simulink model "Copy_of_simulink_ros"  (R2022b)
settings: Solver=FixedStepAuto  StartTime=0.0  StopTime=10.0  FixedStep=0.01  RelTol=1e-3
libraries: robotlib x5
settings Model: Creator=pico  LastModifiedBy=pico

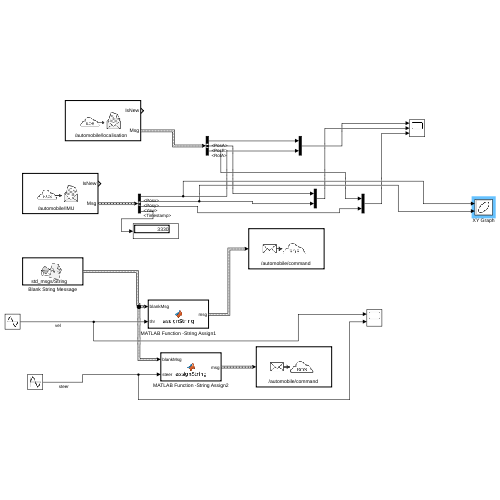
[thumbnail: Simulink's stored preview of the top-level diagram]
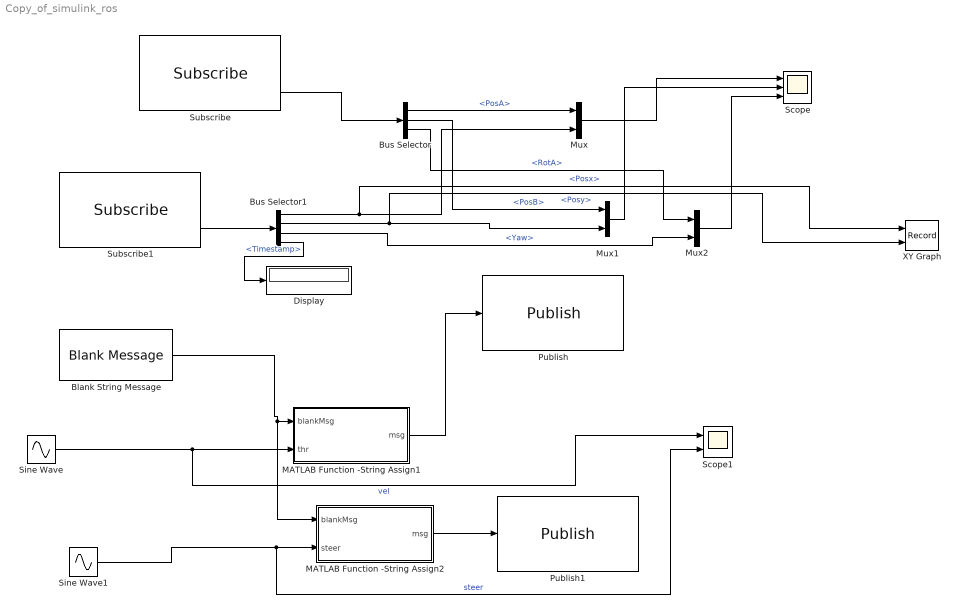
== system Copy_of_simulink_ros ==
  Blank String Message : robotlib/Blank Message  messageClass=Message  entityType=std_msgs/String  messageType=std_msgs/String  SampleTime=inf  legacyBusStruct=off
  Bus Selector : BusSelector  OutputSignals=PosA,PosB,RotA
  Bus Selector1 : BusSelector  OutputSignals=Posx,Posy,Yaw,Timestamp
  Display : Display
  MATLAB Function -String Assign1 : MATLAB Function  TreatAsAtomicUnit=on
  MATLAB Function -String Assign2 : MATLAB Function  TreatAsAtomicUnit=on
  Mux : Mux  Inputs=2
  Mux1 : Mux  Inputs=2
  Mux2 : Mux  Inputs=2
  Publish : robotlib/Publish  topicSource=Select from ROS network  topic=/automobile/command  messageType=std_msgs/String  legacyBusStruct=off  messageQueueLength=1
      settings: LibrarySourceBlock=roslib/ROS/Publish
  Publish1 : robotlib/Publish  topicSource=Select from ROS network  topic=/automobile/command  messageType=std_msgs/String  legacyBusStruct=off  messageQueueLength=1
      settings: LibrarySourceBlock=roslib/ROS/Publish
  Scope : Scope  NumInputPorts=3
  Scope1 : Scope  NumInputPorts=2
  Sine Wave : Sin  Amplitude=2.5  Bias=3  SampleTime=0
  Sine Wave1 : Sin  Amplitude=5  Frequency=2  SampleTime=0
  Subscribe : robotlib/Subscribe  topicSource=Select from ROS network  topic=/automobile/localisation  messageType=utils/localisation  SampleTime=-1  legacyBusStruct=off  messageQueueLength=1
      settings: LibrarySourceBlock=roslib/ROS/Subscribe
  Subscribe1 : robotlib/Subscribe  topicSource=Select from ROS network  topic=/automobile/IMU  messageType=utils/IMU  SampleTime=-1  legacyBusStruct=off  messageQueueLength=1
      settings: LibrarySourceBlock=roslib/ROS/Subscribe
  XY Graph : Record  FileSettingsInternal="{\"entries\":[{\"content\":{\"excelSettings\":{\"content\":{},\"type\":\"Streamout.ExcelSettings\"}},\"type\":\"Streamout.FileSettingStorage\",\"uuid\":\"e51b2920-8d42-452a-b452-2900fad765ce\"}],\"packageUris\":[\"http://schema.mathworks.com/mf0/streamout_blocks/R2020a\"],\"version\":\"1.0\"}"  Layout=[1 1]  SignalsInternal="{\"entries\":[{\"content\":{\"signals\":[{\"content\":{\"blockPath\":[\"simulink_ros/XY Graph\"],\"channel\":[],\"dimensions\":[1],\"domain\":\"simulink_ros/XY Graph\",\"lineColor\":\"#a2142f\",\"plots\":[1],\"port\":1,\"sid\":[\"\"],\"signalID\":1728,\"signalName\":\"<Posx>\"},\"type\":\"RecordBlkView.Signal\",\"uuid\":\"d8332a72-887d-4bf0-9569-057e20747bf9\"},{\"content\":{\"blockPath\":[\"simulink_ros/XY Graph\"],\"channel\":[],\"dimensions\":[1],\"domain\":\"simulink_ros/XY Graph\",\"lineColor\":\"#139fff\",\"plots\":[1],\"port\":2,\"sid\":[\"\"],\"signalID\":1732,\"signalName\":\"<Posy>\"},\"type\":\"RecordBlkView.Signal\",\"uuid\":\"ee58e5d7-22af-4a01-a3d3-c94aa3d0d7b0\"}]},\"type\":\"RecordBlkView.InputSignals\",\"uuid\":\"e0c6eb76-3918-4986-a988-b23fbc1792f6\"}],\"packageUris\":[\"http://schema.mathworks.com/mf0/streamout_blocks/R2020a\"],\"version\":\"1.0\"}"  VisualizationBindings="{\"xyplotplugin\":{\"info\":[{\"series\":[{\"bindingParametersList\":[{\"parameter\":\"X-Axis\",\"signalID\":1728,\"signalName\":\"<Posx>\"},{\"parameter\":\"Y-Axis\",\"signalID\":1732,\"signalName\":\"<Posy>\"}],\"seriesID\":33123}],\"subplotID\":1}]}}"  CompatibilityTag=XY
  wires:
  Subscribe/2 -> Bus Selector/1
  Bus Selector/1 -> Mux/1  "<PosA>"
  Blank String Message/1 -> MATLAB Function -String Assign2/1(blankMsg), MATLAB Function -String Assign1/1(blankMsg)
  MATLAB Function -String Assign1/1(msg) -> Publish/1
  Sine Wave/1 -> Scope1/1, MATLAB Function -String Assign1/2(thr)  "vel"
  MATLAB Function -String Assign2/1(msg) -> Publish1/1
  Sine Wave1/1 -> Scope1/2, MATLAB Function -String Assign2/2(steer)  "steer"
  Subscribe1/2 -> Bus Selector1/1
  Bus Selector1/1 -> XY Graph/1, Mux/2  "<Posx>"
  Bus Selector1/2 -> XY Graph/2, Mux1/2  "<Posy>"
  Mux/1 -> Scope/1
  Bus Selector/2 -> Mux1/1  "<PosB>"
  Mux1/1 -> Scope/2
  Bus Selector1/3 -> Mux2/2  "<Yaw>"
  Bus Selector/3 -> Mux2/1  "<RotA>"
  Mux2/1 -> Scope/3
  Bus Selector1/4 -> Display/1  "<Timestamp>"

== matlab function Copy_of_simulink_ros/MATLAB Function -String Assign2 ==
  data: blankMsg input; msg output Bus: SL_Bus_simulink_ros_std_msgs_String; steer input
function msg = assignString(blankMsg,steer)
% assignString - Assign a string in a ROS message
%
% MSG = assignString(blankMsg) assigns a known string value to a 
%  string field in a ROS message, and outputs the updated ROS message.
%
%  blankMsg (input): A bus for a 'std_msgs/String' message. This is 
%      used to initialize the output. 
%  msg (output): A bus for a 'std_msgs/String' message, with the Data 
%      field set to a string.

%   Copyright 2015 The MathWorks, Inc.
%#codegen

% Note: The datatype of 'msg' has been explicitly set to the appropriate 
% Simulink bus type ("Bus: SL_Bus_robotROSMessageUsageExample_std_msgs_String"). 
%
% If the model name is changed, the datatype needs to be changed as well:
%   1) Click "Edit Data" in the Editor toolstrip to open "Ports and Data Manager"
%   2) Select "msg". From the "Type" dropdown, select "--- Refresh data types ---"
%   3) Set datatype to "Bus: SL_Bus_<modelname>_std_msgs_String"
    
% stringToAssign = 'information';
steer_string = sprintf('%.1f',steer);
% "{\"action\": \"1\", \"speed\": -0.1}"
stringToAssign = ['{"action": "2", "steerAngle": ',steer_string,'}'];%['action\', '1', 'speed',u];

msg = blankMsg;

% msg (std_msgs/String) consists of
%           Data : array of type uint8
%   Data_SL_Info : struct with fields CurrentLength, ReceivedLength
strLength = length(stringToAssign);
msg.Data(1:strLength) = uint8(stringToAssign);
msg.Data_SL_Info.CurrentLength = uint32(strLength);

== matlab function Copy_of_simulink_ros/MATLAB Function -String Assign1 ==
  data: blankMsg input; msg output Bus: SL_Bus_simulink_ros_std_msgs_String; thr input
function msg = assignString(blankMsg,thr)
% assignString - Assign a string in a ROS message
%
% MSG = assignString(blankMsg) assigns a known string value to a 
%  string field in a ROS message, and outputs the updated ROS message.
%
%  blankMsg (input): A bus for a 'std_msgs/String' message. This is 
%      used to initialize the output. 
%  msg (output): A bus for a 'std_msgs/String' message, with the Data 
%      field set to a string.

%   Copyright 2015 The MathWorks, Inc.
%#codegen

% Note: The datatype of 'msg' has been explicitly set to the appropriate 
% Simulink bus type ("Bus: SL_Bus_robotROSMessageUsageExample_std_msgs_String"). 
%
% If the model name is changed, the datatype needs to be changed as well:
%   1) Click "Edit Data" in the Editor toolstrip to open "Ports and Data Manager"
%   2) Select "msg". From the "Type" dropdown, select "--- Refresh data types ---"
%   3) Set datatype to "Bus: SL_Bus_<modelname>_std_msgs_String"
    
thr_string = sprintf('%.1f',thr);
% "{\"action\": \"1\", \"speed\": -0.1}"
stringToAssign = ['{"action": "1", "speed": ',thr_string,'}'];%['action\', '1', 'speed',u];

msg = blankMsg;

% msg (std_msgs/String) consists of
%           Data : array of type uint8
%   Data_SL_Info : struct with fields CurrentLength, ReceivedLength
strLength = length(stringToAssign);
msg.Data(1:strLength) = uint8(stringToAssign);
msg.Data_SL_Info.CurrentLength = uint32(strLength);
